simulink model "shl26df_user_input"  (R2024b)
settings: Solver=VariableStepAuto  StartTime=0.0  StopTime=10  RelTol=1e-3
undefined symbols (not defined in the file): X, Y, Z
libraries: sm_lib x261, nesl_utility x53
(part 1 of 6)
settings Model: Creator=danie  LastModifiedBy=danie
settings ExplorerConfigSet: InternalSimMechanicsExplorerSettings="<ExplorerConfiguration><canonicalview>default</canonicalview><AnimationSetting><BasePlaybackSpeed>1.0</BasePlaybackSpeed><PlaybackSpeedFactor>1.0</PlaybackSpeedFactor></AnimationSetting><TilePanel><TileInfo><Tiles Columns=\"1\" Count=\"1\" Rows=\"1\"><Column Weight=\"1\"/><Row Weight=\"1\"/><Tile Height=\"1\" Width=\"1\" X=\"0\" Y=\"0\"/></Tiles></TileInfo><SceneInfo><SceneViewer><BGColor><R>0.60000002384185791</R><G>0.60000002384185791</G><B>0.60000002384185791</B></BGColor><Camera><DoPerspective>off</DoPerspective><Position><X>1.00422962009906769</X><Y>1.86264514923095703e-09</Y><Z>0.224083766341209856</Z></Position><Center><X>0.00422962009906768799</X><Y>1.86264514923095703e-09</Y><Z>0.224083766341209856</Z></Center><Up><X>-0</X><Y>0</Y><Z>1</Z></Up><ViewLimDist>1</ViewLimDist><YLim>0.230661469101905825</YLim><XLim>0.429980403124147148</XLim></Camera></SceneViewer></SceneInfo></TilePanel><MechEditorPanel><Cameras/><GfxPanelCameraMap/><VideoCreator><PlaybackSpeedRatio>1.0</PlaybackSpeedRatio><FrameRate>30</FrameRate><VideoFormat>Motion JPEG AVI</VideoFormat><FrameSize>auto</FrameSize></VideoCreator></MechEditorPanel></ExplorerConfiguration>"

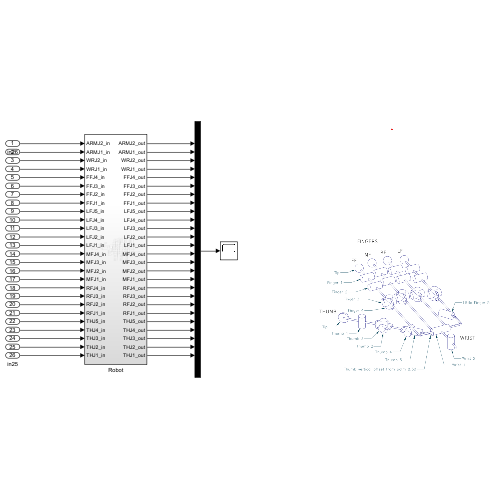
[thumbnail: Simulink's stored preview of the top-level diagram]
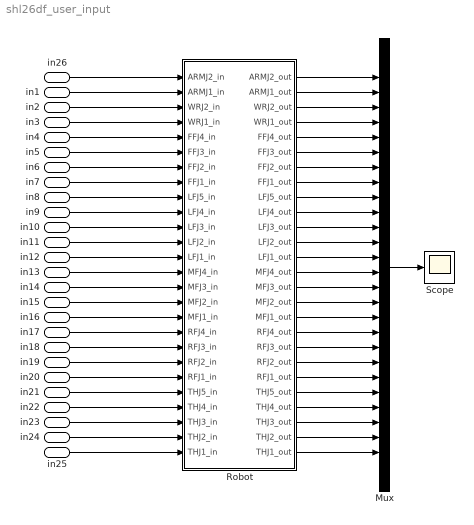
== system shl26df_user_input ==
  in26 : Inport
  in1 : Inport  Port=2
  in2 : Inport  Port=3
  in3 : Inport  Port=4
  in4 : Inport  Port=5
  in5 : Inport  Port=6
  in6 : Inport  Port=7
  in7 : Inport  Port=8
  in8 : Inport  Port=9
  in9 : Inport  Port=10
  in10 : Inport  Port=11
  in11 : Inport  Port=12
  in12 : Inport  Port=13
  in13 : Inport  Port=14
  in14 : Inport  Port=15
  in15 : Inport  Port=16
  in16 : Inport  Port=17
  in17 : Inport  Port=18
  in18 : Inport  Port=19
  in19 : Inport  Port=20
  in20 : Inport  Port=21
  in21 : Inport  Port=22
  in22 : Inport  Port=23
  in23 : Inport  Port=24
  in24 : Inport  Port=25
  in25 : Inport  Port=26
  Mux : Mux  Inputs=26
  Robot : Subsystem
  Scope : Scope
  wires:
  Mux/1 -> Scope/1
  in1/1 -> Robot/2(ARMJ1_in)
  in2/1 -> Robot/3(WRJ2_in)
  in3/1 -> Robot/4(WRJ1_in)
  in4/1 -> Robot/5(FFJ4_in)
  in5/1 -> Robot/6(FFJ3_in)
  in6/1 -> Robot/7(FFJ2_in)
  in7/1 -> Robot/8(FFJ1_in)
  in8/1 -> Robot/9(LFJ5_in)
  in9/1 -> Robot/10(LFJ4_in)
  in10/1 -> Robot/11(LFJ3_in)
  in11/1 -> Robot/12(LFJ2_in)
  in12/1 -> Robot/13(LFJ1_in)
  in13/1 -> Robot/14(MFJ4_in)
  in14/1 -> Robot/15(MFJ3_in)
  in15/1 -> Robot/16(MFJ2_in)
  in16/1 -> Robot/17(MFJ1_in)
  in17/1 -> Robot/18(RFJ4_in)
  in18/1 -> Robot/19(RFJ3_in)
  in19/1 -> Robot/20(RFJ2_in)
  in20/1 -> Robot/21(RFJ1_in)
  in21/1 -> Robot/22(THJ5_in)
  in22/1 -> Robot/23(THJ4_in)
  in23/1 -> Robot/24(THJ3_in)
  in24/1 -> Robot/25(THJ2_in)
  in25/1 -> Robot/26(THJ1_in)
  in26/1 -> Robot/1(ARMJ2_in)
  Robot/1(ARMJ2_out) -> Mux/1
  Robot/2(ARMJ1_out) -> Mux/2
  Robot/3(WRJ2_out) -> Mux/3
  Robot/4(WRJ1_out) -> Mux/4
  Robot/5(FFJ4_out) -> Mux/5
  Robot/6(FFJ3_out) -> Mux/6
  Robot/7(FFJ2_out) -> Mux/7
  Robot/8(FFJ1_out) -> Mux/8
  Robot/9(LFJ5_out) -> Mux/9
  Robot/10(LFJ4_out) -> Mux/10
  Robot/11(LFJ3_out) -> Mux/11
  Robot/12(LFJ2_out) -> Mux/12
  Robot/13(LFJ1_out) -> Mux/13
  Robot/14(MFJ4_out) -> Mux/14
  Robot/15(MFJ3_out) -> Mux/15
  Robot/17(MFJ1_out) -> Mux/17
  Robot/16(MFJ2_out) -> Mux/16
  Robot/18(RFJ4_out) -> Mux/18
  Robot/19(RFJ3_out) -> Mux/19
  Robot/20(RFJ2_out) -> Mux/20
  Robot/21(RFJ1_out) -> Mux/21
  Robot/22(THJ5_out) -> Mux/22
  Robot/23(THJ4_out) -> Mux/23
  Robot/24(THJ3_out) -> Mux/24
  Robot/25(THJ2_out) -> Mux/25
  Robot/26(THJ1_out) -> Mux/26
